simulink model "P2_SIL_Model_Diag"  (R2016a)
settings: Solver=ode2  StartTime=0.0  StopTime=Cycle_End  RelTol=1e-3
undefined symbols (not defined in the file): air, APP1_OOR, APP2_OOR, APP_Conversion_IN, APP_Mismatch, bms_inletair_temp, bms_maxchargecurrent, bms_maxdischargecurrent, BMS_Notfallkuehlung, BPP_Flt, cal, clt, ClutchEngag, CrankRequest, dcdc, eng, Engine, EngOverTemp, ENGTRQ_MSMCH_Degraded_CP, ENGTRQ_MSMCH_ErrCritical_CP, ENGTRQ_MSMCH_LimpHome_CP, EngTrqMismatch, env, ess, ESS, ESSOverTemp, fd, FFD, g, gb, Grade, IMG, KeyPos_Flt, KeyPosition, lib_APP_Conversion_IN, lib_ESS_plant_V1_2, lib_OBC_Manager, LossCAN, max_vehicle_rad_air_flow, MCUOverTemp, mot, MotDirMismatch, MotOverTemp, MotTrqMismatch, mph2kph, mph2ms, NeutralGear, obc, OBC_Manager, ParkGear, PRNDL_Flt, ReverseGear, RFD, rho, ShiftLeverPosition, sigbuilder_block, Speed, t_amb, time, tloop ... (+2)
libraries: simulink x104, EC2_libraries x12, Diagnostic x11, lib_CANerror_Detect x3, Utility x1
(part 9 of 11)

== system P2_SIL_Model_Diag/Controller/HSC/Powertrain Manager/Torque Distribution/Supervisory  Control  Logic1/VehReady.Transition.SyncCtrl ==
  EngSpeed : Inport
  MotorSpeed : Inport  Port=2
  f : TriggerPort  TriggerType=function-call  VariantControl=Variant
      settings: CopyFcn=Stateflow.SLINSF.SimulinkMan.removeBlockPreDeleteFcn  PreDeleteFcn=Stateflow.SLINSF.SimulinkMan.unsafePredeleteFcn
  Kp : Gain  Gain=1/100
  Saturation : Saturate  UpperLimit=20  LowerLimit=0
  Scope : Scope  NumInputPorts=2
  Sum : Sum  Inputs=|+-
  EngApp : Outport
  wires:
  MotorSpeed/1 -> Scope/1, Sum/1  "RPM"
  EngSpeed/1 -> Scope/2, Sum/2
  Sum/1 -> Kp/1
  Kp/1 -> Saturation/1
  Saturation/1 -> EngApp/1

== system P2_SIL_Model_Diag/Controller/HSC/Powertrain Manager/Torque Distribution/Supervisory  Control  Logic1/VehReady.Transition1.SyncCtrl ==
  EngSpeed : Inport
  MotorSpeed : Inport  Port=2
  f : TriggerPort  TriggerType=function-call  VariantControl=Variant
      settings: CopyFcn=Stateflow.SLINSF.SimulinkMan.removeBlockPreDeleteFcn  PreDeleteFcn=Stateflow.SLINSF.SimulinkMan.unsafePredeleteFcn
  Kp : Gain  Gain=1/100
  Saturation : Saturate  UpperLimit=20  LowerLimit=0
  Sum : Sum  Inputs=|+-
  EngApp : Outport
  wires:
  MotorSpeed/1 -> Sum/1  "RPM"
  EngSpeed/1 -> Sum/2
  Sum/1 -> Kp/1
  Kp/1 -> Saturation/1
  Saturation/1 -> EngApp/1

== system P2_SIL_Model_Diag/Controller/HSC/Powertrain Manager/Torque Distribution/Supervisory  Control  Logic1/VehReady.Transition2.SyncCtrl ==
  EngSpeed : Inport
  MotorSpeed : Inport  Port=2
  f : TriggerPort  TriggerType=function-call  VariantControl=Variant
      settings: CopyFcn=Stateflow.SLINSF.SimulinkMan.removeBlockPreDeleteFcn  PreDeleteFcn=Stateflow.SLINSF.SimulinkMan.unsafePredeleteFcn
  Kp : Gain  Gain=1/100
  Saturation : Saturate  UpperLimit=20  LowerLimit=0
  Sum : Sum  Inputs=|+-
  EngApp : Outport
  wires:
  MotorSpeed/1 -> Sum/1  "RPM"
  EngSpeed/1 -> Sum/2
  Sum/1 -> Kp/1
  Kp/1 -> Saturation/1
  Saturation/1 -> EngApp/1

== system P2_SIL_Model_Diag/Controller/HSC/Powertrain Manager/Torque Distribution/SysPwrMd ==
  SysPwrMd : Inport
  EngRunAtv : Inport  Port=2
  EngOnReq : Inport  Port=3
  Constant1 : Constant  Value=3
  Constant2 : Constant
  Saturation2 : Saturate  UpperLimit=2  LowerLimit=0
  Saturation3 : Saturate  UpperLimit=2  LowerLimit=0
  Switch1 : Switch  Threshold=1
  Switch2 : Switch  Threshold=1
  Switch3 : Switch  Threshold=1
  Out1 : Outport
  wires:
  Switch2/1 -> Switch3/3
  Constant1/1 -> Switch1/3
  Constant2/1 -> Switch2/1
  EngRunAtv/1 -> Switch2/2, Switch1/2
  Saturation2/1 -> Switch1/1
  SysPwrMd/1 -> Saturation3/1, Saturation2/1
  Saturation3/1 -> Switch2/3
  EngOnReq/1 -> Switch3/2
  Switch1/1 -> Switch3/1
  Switch3/1 -> Out1/1

== system P2_SIL_Model_Diag/Sensors/CAN/EBCAN/BMS_Antrieb/ISO_Hybrid_01_Resp ==
  Bus Creator : BusCreator  Inputs=3
  Constant : Constant  Value=100
  Constant1 : Constant  Value=100
  Constant2 : Constant  Value=100
  Out1 : Outport
  wires:
  Bus Creator/1 -> Out1/1  "ISO_Hybrid_01_Resp_Data"
  Constant2/1 -> Bus Creator/3  "ISO_Hybrid_01_Resp_Data_byte_5"
  Constant1/1 -> Bus Creator/2  "ISO_Hybrid_01_Resp_Data_byte_4"
  Constant/1 -> Bus Creator/1  "ISO_Hybrid_01_Resp_Data_byte_3"

== system P2_SIL_Model_Diag/Sensors/CAN/EBCAN/BMS_Antrieb/NMH_BMS ==
  In1 : Inport
  Bus Creator : BusCreator  Inputs=5
  Bus Selector : BusSelector  OutputSignals=NMH_BMS_Car_WakeUp,NMH_BMS_Normal_Mode_1,NMH_BMS_Normal_Mode_2,NMH_BMS_Start_1,NMH_BMS_Start_2
  Out1 : Outport
  wires:
  Bus Selector/1 -> Bus Creator/1  "<NMH_BMS_Car_WakeUp>"
  Bus Selector/2 -> Bus Creator/2  "<NMH_BMS_Normal_Mode_1>"
  Bus Selector/3 -> Bus Creator/3  "<NMH_BMS_Normal_Mode_2>"
  Bus Selector/4 -> Bus Creator/4  "<NMH_BMS_Start_1>"
  Bus Selector/5 -> Bus Creator/5  "<NMH_BMS_Start_2>"
  Bus Creator/1 -> Out1/1  "NMH_BMS"
  In1/1 -> Bus Selector/1

== system P2_SIL_Model_Diag/Sensors/CAN/EBCAN/CCM/ISO_Hybrid_01_Resp ==
  Bus Creator : BusCreator  Inputs=3
  Constant : Constant
  Constant1 : Constant
  Constant2 : Constant
  Out1 : Outport
  wires:
  Constant/1 -> Bus Creator/1  "ISO_Hybrid_01_Resp_Data_byte_3"
  Constant1/1 -> Bus Creator/2  "ISO_Hybrid_01_Resp_Data_byte_4"
  Constant2/1 -> Bus Creator/3  "ISO_Hybrid_01_Resp_Data_byte_5"
  Bus Creator/1 -> Out1/1  "ISO_Hybrid_01_Resp_Data"

== system P2_SIL_Model_Diag/Sensors/CAN/EBCAN/CCM/NMH_BMS ==
  Bus Creator : BusCreator  Inputs=5
  Constant{,1..4} (5 alike) : Constant
  Out1 : Outport
  wires:
  Bus Creator/1 -> Out1/1  "NMH_BMS"
  Constant4/1 -> Bus Creator/5  "NMH_BMS_Start_2"
  Constant3/1 -> Bus Creator/4  "NMH_BMS_Start_1"
  Constant2/1 -> Bus Creator/3  "NMH_BMS_Normal_Mode_2"
  Constant1/1 -> Bus Creator/2  "NMH_BMS_Normal_Mode_1"
  Constant/1 -> Bus Creator/1  "NMH_BMS_Car_WakeUp"

== system P2_SIL_Model_Diag/Sensors/CAN/EBCAN/ECM/ETEI_Engine_Torque_Status ==
  In1 : Inport
  Out1 : Outport
  wires:
  In1/1 -> Out1/1  "EngActStdyStTorq"

== system P2_SIL_Model_Diag/Sensors/CAN/EBCAN/ECM/PPEI_Vehicle_Speed_and_Distance ==
  In1 : Inport
  Out1 : Outport
  wires:
  In1/1 -> Out1/1  "VehSpdAvgDrvn"

== system P2_SIL_Model_Diag/Sensors/CAN/HV_CAN/BMS_Hybrid/BMS_HYB_02 ==
  In1 : Inport
  Bus Creator : BusCreator  Inputs=10
  Bus Selector : BusSelector  OutputSignals=BMS_Fehler_HS_offen,BMS_Fehler_Pilot,BMS_Init_abgescholssen,BMS_IstModus,BMS_IstSpannung,BMS_IstStrom,BMS_SleepInd,BMS_Fehler_Isolation,BMS_Fehler_HVBattAbschaltung,MO_BMS_Sollmodus
  Out1 : Outport
  wires:
  Bus Selector/1 -> Bus Creator/1  "<BMS_Fehler_HS_offen>"
  Bus Selector/2 -> Bus Creator/2  "<BMS_Fehler_Pilot>"
  Bus Selector/3 -> Bus Creator/3  "<BMS_Init_abgescholssen>"
  Bus Selector/4 -> Bus Creator/4  "<BMS_IstModus>"
  Bus Selector/5 -> Bus Creator/5  "<BMS_IstSpannung>"
  Bus Selector/6 -> Bus Creator/6  "<BMS_IstStrom>"
  Bus Selector/7 -> Bus Creator/7  "<BMS_SleepInd>"
  Bus Creator/1 -> Out1/1  "BMS_HYB_02"
  In1/1 -> Bus Selector/1
  Bus Selector/8 -> Bus Creator/8  "<BMS_Fehler_Isolation>"
  Bus Selector/9 -> Bus Creator/9  "<BMS_Fehler_HVBattAbschaltung>"
  Bus Selector/10 -> Bus Creator/10  "<MO_BMS_Sollmodus>"

== system P2_SIL_Model_Diag/Sensors/CAN/HV_CAN/BMS_Hybrid/BMS_HYB_03 ==
  In1 : Inport
  Bus Selector : BusSelector  OutputSignals=BMS_SOC
  Out1 : Outport
  wires:
  Bus Selector/1 -> Out1/1  "<BMS_SOC>"
  In1/1 -> Bus Selector/1

== system P2_SIL_Model_Diag/Sensors/CAN/HV_CAN/BMS_Hybrid/BMS_HYB_04 ==
  In1 : Inport
  Bus Selector : BusSelector  OutputSignals=BMS_Spannung_ZwKr
  Out1 : Outport
  wires:
  In1/1 -> Bus Selector/1  "BMS_Spannung_ZwKr"
  Bus Selector/1 -> Out1/1  "<BMS_Spannung_ZwKr>"

== system P2_SIL_Model_Diag/Sensors/CAN/HV_CAN/MCU/M165_Motor_Position_Info ==
  In1 : Inport
  Out1 : Outport
  wires:
  In1/1 -> Out1/1  "D2_Motor_Speed"

== system P2_SIL_Model_Diag/Sensors/CAN/HV_CAN/MCU/M166_Current_Info ==
  In1 : Inport
  Out1 : Outport
  wires:
  In1/1 -> Out1/1  "D4_DC_Bus_Current"

== system P2_SIL_Model_Diag/Sensors/CAN/HV_CAN/MCU/M167_Voltage_Info ==
  In1 : Inport
  Out1 : Outport
  wires:
  In1/1 -> Out1/1  "D1_DC_Bus_Voltage"

== system P2_SIL_Model_Diag/Sensors/CAN/HV_CAN/MCU/M170_Internal_States ==
  In1 : Inport
  Out1 : Outport
  wires:
  In1/1 -> Out1/1  "D6_Inverter_Enable_State"

== system P2_SIL_Model_Diag/Sensors/CAN/HV_CAN/MCU/M172_Torque_And_Timer_Info ==
  In1 : Inport
  Out1 : Outport
  wires:
  In1/1 -> Out1/1  "D2_Torque_Feedback"

== system P2_SIL_Model_Diag/Sensors/CAN/HV_CAN/MCU/M192_Command_Message ==
  In1 : Inport
  Out1 : Outport
  wires:
  In1/1 -> Out1/1  "Torque_Command"

== system P2_SIL_Model_Diag/Sensors/CAN/VEH_CAN/BCM/PPEI_Brake_Apply_Status ==
  In1 : Inport
  Out1 : Outport
  wires:
  In1/1 -> Out1/1  "BrkPdlPos"

== system P2_SIL_Model_Diag/Sensors/CAN/VEH_CAN/BCM/PPEI_Platfrom_General_Status ==
  In1 : Inport
  Out1 : Outport
  wires:
  In1/1 -> Out1/1  "SysPwrMd"

== system P2_SIL_Model_Diag/Sensors/CAN/VEH_CAN/EBCM/PPEI_Chassis_General_Status_1 ==
  Constant : Constant
  Out1 : Outport
  wires:
  Constant/1 -> Out1/1  "BrkPdlDrvAppPrsDetcd"

== system P2_SIL_Model_Diag/Camaro Plant Model/ESS/Soft BMS/Limits/Average Current/60 sec rolling average1 ==
  Instant : Inport
  1 second : Delay  DelayLength=1/tloop  InputProcessing=Inherited  SampleTime=tloop
  1sec trigger : Subsystem
  60 sec average : Subsystem
  Gain1 : Gain  Gain=tloop
  Sum1 : Sum  Inputs=++-
  accumulate : Memory  InheritSampleTime=on
  accumulate1 : Memory  InheritSampleTime=on
  Average : Outport
  wires:
  accumulate1/1 -> Average/1
  60 sec average/1(Average) -> accumulate1/1
  accumulate/1 -> Sum1/1
  1 second/1 -> Sum1/3
  Instant/1 -> Sum1/2, 1 second/1
  Sum1/1 -> Gain1/1, accumulate/1
  1sec trigger/1(Trigger) -> 60 sec average/Enable
  Gain1/1 -> 60 sec average/1(1sec)

== system P2_SIL_Model_Diag/Camaro Plant Model/ESS/Soft BMS/Limits/Average Current/60 sec rolling average2 ==
  Instant : Inport
  1 second : Delay  DelayLength=1/tloop  InputProcessing=Inherited  SampleTime=tloop
  1sec trigger : Subsystem
  60 sec average : Subsystem
  Gain1 : Gain  Gain=tloop
  Sum1 : Sum  Inputs=++-
  accumulate : Memory  InheritSampleTime=on
  accumulate1 : Memory  InheritSampleTime=on
  Average : Outport
  wires:
  Sum1/1 -> accumulate/1, Gain1/1
  Instant/1 -> 1 second/1, Sum1/2
  1 second/1 -> Sum1/3
  accumulate/1 -> Sum1/1
  60 sec average/1(Average) -> accumulate1/1
  accumulate1/1 -> Average/1
  1sec trigger/1(Trigger) -> 60 sec average/Enable
  Gain1/1 -> 60 sec average/1(1sec)

== system P2_SIL_Model_Diag/Camaro Plant Model/ICE Simple1/Engine Plant Modified/Core Engine/EngEfficiency/Divide by Zero Fix ==
  Multiply : Inport
  Divide : Inport  Port=2
  Compare To Zero : simulink/Logic and Bit Operations/Compare To Zero  relop===  OutDataTypeStr=boolean
  Constant1 : Constant  Value=0
  Constant2 : Constant
  Product2 : Product  Inputs=/*  SaturateOnIntegerOverflow=on  InputSameDT=on  OutDataTypeStr=Inherit: Same as first input
  Switch : Switch  Threshold=1
  Switch1 : Switch  Threshold=1
  Output : Outport
  wires:
  Multiply/1 -> Product2/2
  Switch1/1 -> Output/1
  Constant1/1 -> Switch1/1
  Product2/1 -> Switch1/3
  Switch/1 -> Product2/1
  Divide/1 -> Switch/3, Compare To Zero/1
  Constant2/1 -> Switch/1
  Compare To Zero/1 -> Switch1/2, Switch/2

== system P2_SIL_Model_Diag/Camaro Plant Model/IMG/IMG Plant/Clutch/Speed Calculaion/Clutch Accel ==
  y : Inport
  x : Inport  Port=2
  Mux : Mux  Inputs=2
  Switch : Switch  Threshold=0.5  SaturateOnIntegerOverflow=on  InputSameDT=on
  Zero : Constant  Value=0
  Zero check : RelationalOperator  Operator=~=  InputSameDT=on
  divide : Fcn  Expr=u[1]/u[2]
  eps : Constant  Value=eps
  x\y : Outport
  wires:
  Mux/1 -> divide/1
  x/1 -> Mux/1
  divide/1 -> x\y/1
  y/1 -> Zero check/1, Switch/1
  Zero/1 -> Zero check/2
  Zero check/1 -> Switch/2
  Switch/1 -> Mux/2
  eps/1 -> Switch/3

== system P2_SIL_Model_Diag/Camaro Plant Model/IMG/IMG Plant/Clutch/Speed Calculaion/Slip speed integrator ==
  Integrand : Inport
  Control : Inport  Port=2
  Reset value : Inport  Port=3
  Equal? : RelationalOperator  Operator===  InputSameDT=on
  IC : InitialCondition  Value=init
  Integrator : Integrator  ExternalReset=either  InitialConditionSource=external  LimitOutput=on  LowerSaturationLimit=0  AbsoluteTolerance=1e-3
  Switch : Switch  Threshold=0.5  SaturateOnIntegerOverflow=on  InputSameDT=on
  Switch1 : Switch  Threshold=0.5  SaturateOnIntegerOverflow=on  InputSameDT=on
  Zero : Constant  Value=0  OutDataTypeStr=boolean
  Zero1 : Constant  Value=0
  Output : Outport
  wires:
  IC/1 -> Integrator/3
  Integrand/1 -> Switch/1
  Switch/1 -> Integrator/1
  Equal?/1 -> Switch/2, Integrator/2, Switch1/2
  Zero1/1 -> Switch/3
  Zero/1 -> Equal?/2
  Integrator/1 -> Switch1/1
  Reset value/1 -> IC/1, Switch1/3
  Control/1 -> Equal?/1
  Switch1/1 -> Output/1

== system P2_SIL_Model_Diag/Camaro Plant Model/IMG/IMG Plant/Clutch/Speed Calculaion/input shaft free wheeling losses ==
  input shaft speed : Inport
  Constant1 : Constant  Value=0
  Fcn1 : Fcn  Expr=u==0
  Gain1 : Gain  Gain=0.08  SaturateOnIntegerOverflow=on  OutDataTypeStr=Inherit: Same as input  ParamDataTypeStr=Inherit: Same as input
  Switch2 : Switch  Threshold=0.5  SaturateOnIntegerOverflow=on  InputSameDT=on
  input shaft decel : Outport
  wires:
  input shaft speed/1 -> Switch2/3, Fcn1/1
  Fcn1/1 -> Switch2/2
  Gain1/1 -> input shaft decel/1
  Switch2/1 -> Gain1/1
  Constant1/1 -> Switch2/1

== system P2_SIL_Model_Diag/Camaro Plant Model/IMG/IMG Plant/Electric Machine/Calculate Mot Efficiency, MotPwrMech, and, MotPwrElec/Lower Limit ==
  In1 : Inport
  Constant3 : Constant  Value=Lolimit
  MinMax : MinMax  Function=max  Inputs=2
  Out1 : Outport
  wires:
  In1/1 -> MinMax/1
  Constant3/1 -> MinMax/2
  MinMax/1 -> Out1/1

== system P2_SIL_Model_Diag/Camaro Plant Model/IMG/IMG Plant/Electric Machine/MotTrqExcessTrigger/Signal Builder ==
  Demux : Demux  Tag=STV Demux  Outputs=1
  FromWs : FromWorkspace  Tag=STV FromWs  VariableName=tuvar  SampleTime=0
      SigBuilderData=|
      | common.afterFinalStr = 'Extrapolate'
      | common.sampleTime = 0
      | dataSet.timeRange = [0 521]
      | dataSet.name = 'Group 1'
      | sbobj.Groups.Name = 'Group 1'
      | sbobj.Groups.Signals.Name = 'Signal 1'
      | sbobj.Groups.Signals.XData = [0 75 100 220 245 521]
      | sbobj.Groups.Signals.YData = [0 0 0 0 0 0]
      | sbobj.Groups.TimeRange = [0 521]
  Signal 1 : Outport  Tag=STV Outport
  wires:
  Demux/1 -> Signal 1/1
  FromWs/1 -> Demux/1

== system P2_SIL_Model_Diag/Camaro Plant Model/IMG/IMG Plant/Electric Machine/Torque Calculation/electric machine filter ==
  trq : Inport
  Interval Test : simulink/Logic and Bit Operations/Interval Test  IntervalClosedRight=on  uplimit=0.02  IntervalClosedLeft=on  lowlimit=-0.02  OutDataTypeStr=boolean
  Switch : Switch  Threshold=0.5
  electric machine time response : TransferFcn  Denominator=[mot.plant.init.time_response 1]
  filtered : Outport
  wires:
  electric machine time response/1 -> Switch/3
  Interval Test/1 -> Switch/2
  trq/1 -> Interval Test/1, electric machine time response/1, Switch/1
  Switch/1 -> filtered/1

== system P2_SIL_Model_Diag/Camaro Plant Model/IMG/IMG Plant/Electric Machine/Torque Calculation/max torque  ==
  cmd : Inport
  speed : Inport  Port=2
  Memory : Memory
  Peak trq max - Motoring : Lookup  InputValues=mot.plant.init.regen.trq_max.idx1_spd  Table=mot.plant.init.motor.trq_max.map  LookUpMeth=Interpolation-Use End Values  SaturateOnIntegerOverflow=on
  Peak trq max - Regen : Lookup  InputValues=mot.plant.init.regen.trq_max.idx1_spd  Table=mot.plant.init.regen.trq_max.map  LookUpMeth=Interpolation-Use End Values  SaturateOnIntegerOverflow=on
  Switch1 : Switch  SaturateOnIntegerOverflow=on
  rad/s  to RPM : Gain  Gain=30/pi
  max torque : Outport
  wires:
  Peak trq max - Regen/1 -> Switch1/3
  Peak trq max - Motoring/1 -> Switch1/1
  speed/1 -> rad/s  to RPM/1
  cmd/1 -> Switch1/2
  Switch1/1 -> max torque/1
  Memory/1 -> Peak trq max - Motoring/1, Peak trq max - Regen/1
  rad/s  to RPM/1 -> Memory/1

== system P2_SIL_Model_Diag/Camaro Plant Model/IMG/Soft MCU/Torque Calculation/max torque /Divide by zero ==
  In1 : Inport
  Compare To Constant : simulink/Logic and Bit Operations/Compare To Constant  relop===  const=0  OutDataTypeStr=boolean
  Constant1 : Constant
  Switch2 : Switch  Criteria=u2 > Threshold
  Out1 : Outport
  wires:
  Constant1/1 -> Switch2/1
  Compare To Constant/1 -> Switch2/2
  In1/1 -> Switch2/3, Compare To Constant/1
  Switch2/1 -> Out1/1

== system P2_SIL_Model_Diag/Camaro Plant Model/IMG/Soft MCU/Torque Calculation/max torque /Heat index ==
  note: Heat index calculation
  cont torque : Inport
  torque : Inport  Port=2
  Abs : Abs  SaturateOnIntegerOverflow=on
  Divide : Subsystem  mask(Divide){}
      mask Display: disp('Divide')
  Heat Energy Factor : Integrator  InitialCondition=-0.3  LimitOutput=on  UpperSaturationLimit=1  LowerSaturationLimit=-0.3
  Heating Constant : Gain  Gain=0.3/mot.plant.init.t_max_trq  SaturateOnIntegerOverflow=on  OutDataTypeStr=Inherit: Same as input  ParamDataTypeStr=Inherit: Same as input
  Saturation : Saturate  UpperLimit=1  LowerLimit=0
  Sum : Sum  Inputs=+-  SaturateOnIntegerOverflow=on  InputSameDT=on  OutDataTypeStr=Inherit: Same as first input
  motor inertia (Nms^2\rad)5 : Constant
  Heat index : Outport
  wires:
  cont torque/1 -> Divide/2(denominator)
  Abs/1 -> Sum/1
  Saturation/1 -> Heat index/1
  motor inertia (Nms^2\rad)5/1 -> Sum/2
  Divide/1(quotient) -> Abs/1
  Sum/1 -> Heating Constant/1
  Heating Constant/1 -> Heat Energy Factor/1
  Heat Energy Factor/1 -> Saturation/1
  torque/1 -> Divide/1(numerator)

== system P2_SIL_Model_Diag/Camaro Plant Model/Transmission1/Transmission Plant/Gearbox/Speed Calculation/P//N ==
  torque input : Inport
  Inertia Input : Inport  Port=2
  gear : Inport  Port=3
  inital speed : Inport  Port=4
  (0,inf) : Saturate  UpperLimit=inf  LowerLimit=0
  Fcn2 : Fcn  Expr=u==0
  Integrator : Integrator  ExternalReset=rising  InitialConditionSource=external
  Memory : Memory
  Subsystem2 : Subsystem
      mask Display: disp('divider')
  Sum : Sum  Inputs=-+|  SaturateOnIntegerOverflow=on  InputSameDT=on  OutDataTypeStr=Inherit: Same as first input
  input shaft free wheeling losses : Subsystem
  speed : Outport
  wires:
  Inertia Input/1 -> Subsystem2/2(In2)
  Fcn2/1 -> Integrator/2
  Subsystem2/1(Out1) -> Integrator/1
  Memory/1 -> Integrator/3
  (0,inf)/1 -> speed/1
  gear/1 -> Fcn2/1
  inital speed/1 -> Memory/1
  torque input/1 -> Sum/2
  Sum/1 -> Subsystem2/1(In1)
  input shaft free wheeling losses/1(input shaft decel) -> Sum/1
  Integrator/1 -> input shaft free wheeling losses/1(input shaft speed), (0,inf)/1

== system P2_SIL_Model_Diag/Camaro Plant Model/Transmission1/Transmission Plant/Gearbox/Speed Calculation/R//D ==
  spd in : Inport
  gear number : Inport  Port=2
  Constant5 : Constant
  Constant6 : Constant  Value=gb.plant.init.shift_time
  Integrator : Integrator  ExternalReset=rising
  Relational Operator4 : RelationalOperator  Operator=~=  InputSameDT=on
  Relational Operator5 : RelationalOperator  Operator=<=  InputSameDT=on
  S-R Flip-Flop : Subsystem  mask(SRFlipFlop){initial_condition=0}
      mask prompts: initial_condition "Initial condition:"
      mask help: S-R Flip Flop Block
  Switch : Switch  Threshold=0.5  SaturateOnIntegerOverflow=on  InputSameDT=on
  Transfer Fcn : TransferFcn  Denominator=[.2 1]
  Unit Delay7 : Memory
  term2 : Terminator
  spd in filtered : Outport
  wires:
  Transfer Fcn/1 -> Switch/1
  Switch/1 -> spd in filtered/1
  Relational Operator5/1 -> S-R Flip-Flop/2(R)
  S-R Flip-Flop/1(Q) -> Switch/2
  Integrator/1 -> Relational Operator5/2
  Relational Operator4/1 -> S-R Flip-Flop/1(S), Integrator/2
  Unit Delay7/1 -> Relational Operator4/2
  S-R Flip-Flop/2(!Q) -> term2/1
  Constant6/1 -> Relational Operator5/1
  Constant5/1 -> Integrator/1
  spd in/1 -> Transfer Fcn/1, Switch/3
  gear number/1 -> Unit Delay7/1, Relational Operator4/1

== system P2_SIL_Model_Diag/Camaro Plant Model/Transmission1/Transmission Plant/Gearbox/Torque calculation/Blending (state dependent) ==
  Input : Inport
  Control (state) : Inport  Port=2
  Linear spline : Fcn  Expr=(u<xl)*yl + (xl<=u)*(u<xc)*((yc-yl)*(u-xl)/(xc-xl)+yl) + (xc<=u)*(u<xr)*((yc-yr)*(u-xr)/(xc-xr)+yr) + (xr<=u)*yr
  Product2 : Product  SaturateOnIntegerOverflow=on  InputSameDT=on  OutDataTypeStr=Inherit: Same as first input
  Output : Outport
  wires:
  Control (state)/1 -> Linear spline/1
  Product2/1 -> Output/1
  Linear spline/1 -> Product2/2
  Input/1 -> Product2/1

== system P2_SIL_Model_Diag/Camaro Plant Model/Transmission1/Transmission Plant/Torque Converter/Speed Calculation/Pump Accel ==
  y : Inport
  x : Inport  Port=2
  Mux : Mux  Inputs=2
  Switch : Switch  Threshold=0.5  SaturateOnIntegerOverflow=on  InputSameDT=on
  Zero : Constant  Value=0
  Zero check : RelationalOperator  Operator=~=  InputSameDT=on
  divide : Fcn  Expr=u[1]/u[2]
  eps : Constant  Value=eps
  x\y : Outport
  wires:
  eps/1 -> Switch/3
  Switch/1 -> Mux/2
  Zero check/1 -> Switch/2
  Zero/1 -> Zero check/2
  y/1 -> Switch/1, Zero check/1
  divide/1 -> x\y/1
  x/1 -> Mux/1
  Mux/1 -> divide/1

== system P2_SIL_Model_Diag/Camaro Plant Model/Transmission1/Transmission Plant/Torque Converter/Speed Calculation/Slip speed integrator ==
  note: torque converter locked => spd in = spd out
      | when unlocked, spd in = integral of (Tin-Tloss)\J
  Integral : Inport
  Control : Inport  Port=2
  Reset value : Inport  Port=3
  Equal? : RelationalOperator  Operator===  OutDataTypeStr=boolean  InputSameDT=on
  IC : InitialCondition  Value=init
  Integrator : Integrator  ExternalReset=either  InitialConditionSource=external  LimitOutput=on  LowerSaturationLimit=0  AbsoluteTolerance=1e-3
  Switch : Switch  Threshold=0.5  SaturateOnIntegerOverflow=on  InputSameDT=on
  Switch1 : Switch  Threshold=0.5  SaturateOnIntegerOverflow=on  InputSameDT=on
  Zero : Constant  Value=0  OutDataTypeStr=boolean
  Zero1 : Constant  Value=0
  Output : Outport
  wires:
  Reset value/1 -> Switch1/3, IC/1
  Switch1/1 -> Output/1
  Integrator/1 -> Switch1/1
  Zero/1 -> Equal?/2
  Zero1/1 -> Switch/3
  Equal?/1 -> Switch1/2, Integrator/2, Switch/2
  Switch/1 -> Integrator/1
  Integral/1 -> Switch/1
  Control/1 -> Equal?/1
  IC/1 -> Integrator/3

== system P2_SIL_Model_Diag/Camaro Plant Model/Transmission1/Transmission Plant/Torque Converter/Torque Calculation/ Hydraulic Dynamic Torque ==
  input_trq : Inport
  Rt : Inport  Port=2
  Rw : Inport  Port=3
  impeller_spd : Inport  Port=4
  Divide : Product  Inputs=*/
  K Factor : Lookup  InputValues=tc.plant.init.k_factor.idx1_spd_ratio  Table=tc.plant.init.k_factor.map  LookUpMeth=Interpolation-Use End Values  SaturateOnIntegerOverflow=on
  Product1 : Product  SaturateOnIntegerOverflow=on  InputSameDT=on  OutDataTypeStr=Inherit: Same as first input
  Product2 : Product  SaturateOnIntegerOverflow=on  InputSameDT=on  OutDataTypeStr=Inherit: Same as first input
  Product3 : Product  SaturateOnIntegerOverflow=on  InputSameDT=on  OutDataTypeStr=Inherit: Same as first input
  Sum : Sum  Inputs=-+
  turbine_trq : Outport
  impeller_trq : Outport  Port=2
  wires:
  Product1/1 -> Divide/2  "K^2"
  Product3/1 -> turbine_trq/1  "Tt_hd"
  Rt/1 -> Product3/1
  input_trq/1 -> Sum/2
  Sum/1 -> impeller_trq/1
  impeller_spd/1 -> Product2/2, Product2/1
  Product2/1 -> Divide/1  "Wi^2"
  Divide/1 -> Product3/2, Sum/1  "Ti_hd"
  K Factor/1 -> Product1/1, Product1/2  "K"
  Rw/1 -> K Factor/1

== system P2_SIL_Model_Diag/Camaro Plant Model/Transmission1/Transmission Plant/Torque Converter/Torque Calculation/spd and trq ratio ==
  impeller spd : Inport
  turbine spd : Inport  Port=2
  Torque Ratio : Lookup  InputValues=tc.plant.init.spd_ratio  Table=tc.plant.init.trq_ratio  LookUpMeth=Interpolation-Use End Values  SaturateOnIntegerOverflow=on
  speed ratio : Subsystem  mask(Divider){}
      mask help: Divide input 1 by input 2.
      mask Help:
      | This block implements a divider; division by zero is taken care of in the following manner:
      | if u[2] equals 0,
      |    the output is u[1]/eps,
      | else
      |    the output is u[1]/u[2].
      mask Display: disp('/')
  Rt : Outport
  Rw : Outport  Port=2
  wires:
  Torque Ratio/1 -> Rt/1
  speed ratio/1(quotient) -> Rw/1, Torque Ratio/1
  impeller spd/1 -> speed ratio/2(denominator)
  turbine spd/1 -> speed ratio/1(numerator)

== system P2_SIL_Model_Diag/Controller/HSC/Camaro Fault Detection/Component Diagnostic/Engine Component Diagnostic/Override  engTrqCmd ==
  note: This subsystem is used to override the model value of a signal to a constant value
  note: Override Switch Subsystem
  In1 : Inport
  Constant : Constant  Value=50
  Multiport Switch : MultiPortSwitch  DataPortOrder=Zero-based contiguous  Inputs=2  zeroidx=on
  Signal Override Switch 0 = Use Model 1 = Use Constant : Constant
  Out1 : Outport
  wires:
  Signal Override Switch 0 = Use Model 1 = Use Constant/1 -> Multiport Switch/1
  In1/1 -> Multiport Switch/2
  Multiport Switch/1 -> Out1/1
  Constant/1 -> Multiport Switch/3

== system P2_SIL_Model_Diag/Controller/HSC/Camaro Fault Detection/Component Diagnostic/Engine Component Diagnostic/TorqMismatch Detection ==
  In1 : Inport
  In2 : Inport  Port=2
  In3 : Inport  Port=3
  Abs : Abs
  Add : Sum  Inputs=+-
  Bus Creator : BusCreator  Inputs=3
  Constant : Constant  Value=cal.ENGTRQ_MSMCH.ErrCritical_CP
  Constant1 : Constant  Value=50
  Constant2 : Constant  Value=cal.ENGTRQ_MSMCH.Degraded_CP
  Constant3 : Constant  Value=cal.ENGTRQ_MSMCH.LimpHome_CP
  Relational Operator : RelationalOperator  OutDataTypeStr=boolean
  Relational Operator1 : RelationalOperator  Operator=>  OutDataTypeStr=boolean
  Relational Operator2 : RelationalOperator  Operator=>  OutDataTypeStr=boolean
  Switch : Switch  Threshold=1
  Terminator : Terminator
  Unit Delay : UnitDelay  Commented=through  SampleTime=-1
  Unit Delay1 : UnitDelay  Commented=through  SampleTime=-1
  "Zero " : Constant  Value=0
  Eng_Torque_Mismch : Outport
  wires:
  In1/1 -> Unit Delay/1
  In2/1 -> Unit Delay1/1
  "Zero "/1 -> Switch/3
  In3/1 -> Switch/2
  Unit Delay/1 -> Add/1
  Constant/1 -> Relational Operator/2
  Add/1 -> Abs/1
  Relational Operator/1 -> Switch/1
  Switch/1 -> Bus Creator/1, Relational Operator2/1, Relational Operator1/1  "Eng_Torque_Mismch_Critical"
  Constant2/1 -> Relational Operator1/2
  Constant3/1 -> Relational Operator2/2
  Relational Operator1/1 -> Bus Creator/2  "Eng_Torque_Mismch_Degrad"
  Relational Operator2/1 -> Bus Creator/3  "Eng_Torque_Mismch_Limp"
  Bus Creator/1 -> Eng_Torque_Mismch/1
  Unit Delay1/1 -> Add/2
  Abs/1 -> Terminator/1
  Constant1/1 -> Relational Operator/1

== system P2_SIL_Model_Diag/Controller/HSC/Camaro Fault Detection/Component Diagnostic/Motor Component Diagnostic/MCU_ESS_Voltage_Mismatch ==
  MCU_Voltage : Inport
  ESS_Voltage : Inport  Port=2
  Abs : Abs
  Add : Sum  Inputs=-+
  Constant : Constant  Value=cal.Diag.MCU.ESSVLT_MSMCH
  Relational Operator : RelationalOperator  OutDataTypeStr=boolean
  MCU_ESS_Voltage_Mismch : Outport
  wires:
  Relational Operator/1 -> MCU_ESS_Voltage_Mismch/1
  Constant/1 -> Relational Operator/2
  Abs/1 -> Relational Operator/1
  ESS_Voltage/1 -> Add/2
  Add/1 -> Abs/1
  MCU_Voltage/1 -> Add/1

== system P2_SIL_Model_Diag/Controller/HSC/Camaro Fault Detection/Component Diagnostic/Motor Component Diagnostic/Motor_Direction_Mismatch ==
  note: 1: mismatch
      | 0: no failure
  Direction_Command : Inport
  Direction_Feedback : Inport  Port=2
  Inverter_enable_state : Inport  Port=3
  Logical Operator : Logic  AllPortsSameDT=off  OutDataTypeStr=boolean
  Relational Operator : RelationalOperator  Operator=~=  OutDataTypeStr=boolean
  Direction_Mismch : Outport
  wires:
  Relational Operator/1 -> Logical Operator/1
  Logical Operator/1 -> Direction_Mismch/1
  Direction_Command/1 -> Relational Operator/1  "Direction_Command"
  Direction_Feedback/1 -> Relational Operator/2  "Direction_Feedback"
  Inverter_enable_state/1 -> Logical Operator/2  "Inverter_enable_state"

== system P2_SIL_Model_Diag/Controller/HSC/Camaro Fault Detection/Component Diagnostic/Motor Component Diagnostic/Override  fault ==
  note: This subsystem is used to override the model value of a signal to a constant value
  note: Override Switch Subsystem
  In1 : Inport
  Multiport Switch : MultiPortSwitch  DataPortOrder=Zero-based contiguous  Inputs=2  zeroidx=on
  Override Value : Constant  Value=0  OutDataTypeStr=double
  Signal Override Switch 0 = Use Model 1 = Use Constant : Constant
  Out1 : Outport
  wires:
  Signal Override Switch 0 = Use Model 1 = Use Constant/1 -> Multiport Switch/1
  In1/1 -> Multiport Switch/2
  Multiport Switch/1 -> Out1/1
  Override Value/1 -> Multiport Switch/3

== system P2_SIL_Model_Diag/Controller/HSC/Camaro Fault Detection/Component Diagnostic/Motor Component Diagnostic/Override  fault1 ==
  note: Override Switch Subsystem
  note: This subsystem is used to override the model value of a signal to a constant value
  In1 : Inport
  Multiport Switch : MultiPortSwitch  DataPortOrder=Zero-based contiguous  Inputs=2  zeroidx=on
  Override Value : Constant  Value=0  OutDataTypeStr=double
  Signal Override Switch 0 = Use Model 1 = Use Constant : Constant  Value=0
  Out1 : Outport
  wires:
  Override Value/1 -> Multiport Switch/3
  Multiport Switch/1 -> Out1/1
  In1/1 -> Multiport Switch/2
  Signal Override Switch 0 = Use Model 1 = Use Constant/1 -> Multiport Switch/1

== system P2_SIL_Model_Diag/Controller/HSC/Camaro Fault Detection/Component Diagnostic/Motor Component Diagnostic/Torque_Mismatch ==
  MCU_torq_command : Inport
  Torq_feedback : Inport  Port=2
  Abs : Abs
  Abs1 : Abs
  Abs2 : Abs
  Add : Sum  Inputs=+-
  Bus Creator : BusCreator  Inputs=3
  Constant : Constant  Value=cal.MOTTRQ_MSMCH.ErrCritical_CP
  Constant1 : Constant  Value=cal.MOTTRQ_MSMCH.Degraded_CP
  Constant2 : Constant  Value=cal.MOTTRQ_MSMCH.LimpHome_CP
  Constant3 : Constant  Value=0
  Conversion  APP1 (%) : DataTypeConversion  OutDataTypeStr=boolean
  Latch : Subsystem
  Relational Operator : RelationalOperator  Operator=>  OutDataTypeStr=boolean
  Relational Operator1 : RelationalOperator  Operator=>  OutDataTypeStr=boolean
  Relational Operator2 : RelationalOperator  Operator=>  OutDataTypeStr=boolean
  Unit Delay : UnitDelay  SampleTime=-1
  MCU_Torque_Mismch : Outport
  wires:
  Unit Delay/1 -> Abs/1
  Abs/1 -> Add/1
  Torq_feedback/1 -> Abs1/1
  Abs1/1 -> Add/2
  MCU_torq_command/1 -> Unit Delay/1
  Constant/1 -> Relational Operator/2
  Constant1/1 -> Relational Operator1/2
  Constant2/1 -> Relational Operator2/2
  Relational Operator1/1 -> Bus Creator/2  "MCU_Torque_Mismch_Degrad"
  Relational Operator2/1 -> Bus Creator/3  "MCU_Torque_Mismch_Limp"
  Bus Creator/1 -> MCU_Torque_Mismch/1
  Add/1 -> Abs2/1
  Abs2/1 -> Relational Operator/1, Relational Operator2/1, Relational Operator1/1
  Constant3/1 -> Conversion  APP1 (%)/1
  Relational Operator/1 -> Latch/1(In1)  "MCU_Torque_Mismch_Critical"
  Latch/1(Out1) -> Bus Creator/1  "MCU_Torque_Mismch_Critical"
  Conversion  APP1 (%)/1 -> Latch/2(In2)

== system P2_SIL_Model_Diag/Controller/HSC/Camaro Fault Detection/Input Conversions/BMS_Conversions/BMS_rollingAliveCnt ==
  Constant : Constant
  Rolling Alive Counter : Stateflow chart  TreatAsAtomicUnit=on
  Switch : Switch  Criteria=u2 > Threshold
  Out1 : Outport
  wires:
  Switch/1 -> Out1/1  "BMS_rollingAliveCnt [0 1 2 3]"
  [BMS_CAN_fault] -> Switch/2
  Constant/1 -> Switch/1
  Rolling Alive Counter/1(RollingAliveCnt) -> Switch/3

== system P2_SIL_Model_Diag/Controller/HSC/Camaro Fault Detection/Input Conversions/BMS_Conversions/Override  BMS_gdf 0_1 ==
  note: Override Switch Subsystem
  note: This subsystem is used to override the model value of a signal to a constant value
  In1 : Inport
  Multiport Switch : MultiPortSwitch  DataPortOrder=Zero-based contiguous  Inputs=2  zeroidx=on
  Override Value : Constant  Value=0  OutDataTypeStr=double
  Signal Override Switch 0 = Use Model 1 = Use Constant : Constant
  Out1 : Outport
  wires:
  Override Value/1 -> Multiport Switch/3
  Multiport Switch/1 -> Out1/1
  In1/1 -> Multiport Switch/2
  Signal Override Switch 0 = Use Model 1 = Use Constant/1 -> Multiport Switch/1

== system P2_SIL_Model_Diag/Controller/HSC/Camaro Fault Detection/Input Conversions/BMS_Conversions/Override  closeContactorsCmd ==
  note: This subsystem is used to override the model value of a signal to a constant value
  note: Override Switch Subsystem
  In1 : Inport
  Multiport Switch : MultiPortSwitch  DataPortOrder=Zero-based contiguous  Inputs=2  zeroidx=on
  Override Value : Constant  Value=0  OutDataTypeStr=double
  Signal Override Switch 0 = Use Model 1 = Use Constant : Constant  Value=0
  Out1 : Outport
  wires:
  Signal Override Switch 0 = Use Model 1 = Use Constant/1 -> Multiport Switch/1
  In1/1 -> Multiport Switch/2
  Multiport Switch/1 -> Out1/1
  Override Value/1 -> Multiport Switch/3

== system P2_SIL_Model_Diag/Controller/HSC/Camaro Fault Detection/Input Conversions/BMS_Conversions/Override  contactorsClsd ==
  note: This subsystem is used to override the model value of a signal to a constant value
  note: Override Switch Subsystem
  In1 : Inport
  Multiport Switch : MultiPortSwitch  DataPortOrder=Zero-based contiguous  Inputs=2  zeroidx=on
  Override Value : Constant  Value=0  OutDataTypeStr=double
  Signal Override Switch 0 = Use Model 1 = Use Constant : Constant  Value=0
  Out1 : Outport
  wires:
  Signal Override Switch 0 = Use Model 1 = Use Constant/1 -> Multiport Switch/1
  In1/1 -> Multiport Switch/2
  Multiport Switch/1 -> Out1/1
  Override Value/1 -> Multiport Switch/3

== system P2_SIL_Model_Diag/Controller/HSC/Camaro Fault Detection/Input Conversions/BMS_Conversions/Override  essCur_A ==
  note: Override Switch Subsystem
  note: This subsystem is used to override the model value of a signal to a constant value
  In1 : Inport
  Multiport Switch : MultiPortSwitch  DataPortOrder=Zero-based contiguous  Inputs=2  zeroidx=on
  Override Value : Constant  Value=0  OutDataTypeStr=double
  Signal Override Switch 0 = Use Model 1 = Use Constant : Constant  Value=0
  Out1 : Outport
  wires:
  Override Value/1 -> Multiport Switch/3
  Multiport Switch/1 -> Out1/1
  In1/1 -> Multiport Switch/2
  Signal Override Switch 0 = Use Model 1 = Use Constant/1 -> Multiport Switch/1

== system P2_SIL_Model_Diag/Controller/HSC/Camaro Fault Detection/Input Conversions/BMS_Conversions/Override  essSOC_0_1 ==
  note: This subsystem is used to override the model value of a signal to a constant value
  note: Override Switch Subsystem
  In1 : Inport
  Multiport Switch : MultiPortSwitch  DataPortOrder=Zero-based contiguous  Inputs=2  zeroidx=on
  Override Value : Constant  Value=0  OutDataTypeStr=double
  Signal Override Switch 0 = Use Model 1 = Use Constant : Constant  Value=0
  Out1 : Outport
  wires:
  Signal Override Switch 0 = Use Model 1 = Use Constant/1 -> Multiport Switch/1
  In1/1 -> Multiport Switch/2
  Multiport Switch/1 -> Out1/1
  Override Value/1 -> Multiport Switch/3

== system P2_SIL_Model_Diag/Controller/HSC/Camaro Fault Detection/Input Conversions/BMS_Conversions/Override  essTemp_C ==
  note: This subsystem is used to override the model value of a signal to a constant value
  note: Override Switch Subsystem
  In1 : Inport
  Multiport Switch : MultiPortSwitch  DataPortOrder=Zero-based contiguous  Inputs=2  zeroidx=on
  Override Value : Constant  Value=0  OutDataTypeStr=double
  Signal Override Switch 0 = Use Model 1 = Use Constant : Constant
  Out1 : Outport
  wires:
  Signal Override Switch 0 = Use Model 1 = Use Constant/1 -> Multiport Switch/1
  In1/1 -> Multiport Switch/2
  Multiport Switch/1 -> Out1/1
  Override Value/1 -> Multiport Switch/3

== system P2_SIL_Model_Diag/Controller/HSC/Camaro Fault Detection/Input Conversions/BMS_Conversions/Override  hvBattVolt_V ==
  note: This subsystem is used to override the model value of a signal to a constant value
  note: Override Switch Subsystem
  In1 : Inport
  Multiport Switch : MultiPortSwitch  DataPortOrder=Zero-based contiguous  Inputs=2  zeroidx=on
  Override Value : Constant  Value=0  OutDataTypeStr=double
  Signal Override Switch 0 = Use Model 1 = Use Constant : Constant  Value=0
  Out1 : Outport
  wires:
  Signal Override Switch 0 = Use Model 1 = Use Constant/1 -> Multiport Switch/1
  In1/1 -> Multiport Switch/2
  Multiport Switch/1 -> Out1/1
  Override Value/1 -> Multiport Switch/3

== system P2_SIL_Model_Diag/Controller/HSC/Camaro Fault Detection/Input Conversions/BMS_Conversions/Override  hvBusVolt_V ==
  note: Override Switch Subsystem
  note: This subsystem is used to override the model value of a signal to a constant value
  In1 : Inport
  Multiport Switch : MultiPortSwitch  DataPortOrder=Zero-based contiguous  Inputs=2  zeroidx=on
  Override Value : Constant  Value=0  OutDataTypeStr=double
  Signal Override Switch 0 = Use Model 1 = Use Constant : Constant  Value=0
  Out1 : Outport
  wires:
  Override Value/1 -> Multiport Switch/3
  Multiport Switch/1 -> Out1/1
  In1/1 -> Multiport Switch/2
  Signal Override Switch 0 = Use Model 1 = Use Constant/1 -> Multiport Switch/1

== system P2_SIL_Model_Diag/Controller/HSC/Camaro Fault Detection/Input Conversions/BMS_Conversions/Override  rollingAliveCnt [1_3] ==
  note: Override Switch Subsystem
  note: This subsystem is used to override the model value of a signal to a constant value
  In1 : Inport
  Multiport Switch : MultiPortSwitch  DataPortOrder=Zero-based contiguous  Inputs=2  zeroidx=on
  Override Value : Constant  Value=0  OutDataTypeStr=double
  Signal Override Switch 0 = Use Model 1 = Use Constant : Constant  Value=0
  Out1 : Outport
  wires:
  Override Value/1 -> Multiport Switch/3
  Multiport Switch/1 -> Out1/1
  In1/1 -> Multiport Switch/2
  Signal Override Switch 0 = Use Model 1 = Use Constant/1 -> Multiport Switch/1

== system P2_SIL_Model_Diag/Controller/HSC/Camaro Fault Detection/Input Conversions/Clutch_Conversions/Clutch_Rolling ==
  Constant8 : Constant
  Rolling Alive Counter1 : Stateflow chart  TreatAsAtomicUnit=on
  Switch1 : Switch  Criteria=u2 > Threshold
  Out1 : Outport
  wires:
  [Clutch_CAN_fault] -> Switch1/2
  Rolling Alive Counter1/1(RollingAliveCnt) -> Switch1/3
  Constant8/1 -> Switch1/1
  Switch1/1 -> Out1/1  "ClutchRollingAliveCnt [0 1 2 3]"

== system P2_SIL_Model_Diag/Controller/HSC/Camaro Fault Detection/Input Conversions/Clutch_Conversions/Override  Engage_Clutch  ==
  note: This subsystem is used to override the model value of a signal to a constant value
  note: Override Switch Subsystem
  In1 : Inport
  Multiport Switch : MultiPortSwitch  DataPortOrder=Zero-based contiguous  Inputs=2  zeroidx=on
  Override Value : Constant  Value=0  OutDataTypeStr=double
  Signal Override Switch 0 = Use Model 1 = Use Constant : Constant
  Out1 : Outport
  wires:
  Signal Override Switch 0 = Use Model 1 = Use Constant/1 -> Multiport Switch/1
  In1/1 -> Multiport Switch/2
  Multiport Switch/1 -> Out1/1
  Override Value/1 -> Multiport Switch/3

== system P2_SIL_Model_Diag/Controller/HSC/Camaro Fault Detection/Input Conversions/Clutch_Conversions/Override  rollingAliveCnt [123] ==
  note: Override Switch Subsystem
  note: This subsystem is used to override the model value of a signal to a constant value
  In1 : Inport
  Multiport Switch : MultiPortSwitch  DataPortOrder=Zero-based contiguous  Inputs=2  zeroidx=on
  Override Value : Constant  Value=0  OutDataTypeStr=double
  Signal Override Switch 0 = Use Model 1 = Use Constant : Constant  Value=0
  Out1 : Outport
  wires:
  Override Value/1 -> Multiport Switch/3
  Multiport Switch/1 -> Out1/1
  In1/1 -> Multiport Switch/2
  Signal Override Switch 0 = Use Model 1 = Use Constant/1 -> Multiport Switch/1

== system P2_SIL_Model_Diag/Controller/HSC/Camaro Fault Detection/Input Conversions/DriverInput_Conversions/Override  KeyPos [0_3] ==
  note: Override Switch Subsystem
  note: This subsystem is used to override the model value of a signal to a constant value
  In1 : Inport
  Multiport Switch : MultiPortSwitch  DataPortOrder=Zero-based contiguous  Inputs=2  zeroidx=on
  Override Value : Constant  Value=0  OutDataTypeStr=double
  Signal Override Switch 0 = Use Model 1 = Use Constant : Constant  Value=0
  Out1 : Outport
  wires:
  Override Value/1 -> Multiport Switch/3
  Multiport Switch/1 -> Out1/1
  In1/1 -> Multiport Switch/2
  Signal Override Switch 0 = Use Model 1 = Use Constant/1 -> Multiport Switch/1

== system P2_SIL_Model_Diag/Controller/HSC/Camaro Fault Detection/Input Conversions/DriverInput_Conversions/Override APP (%) ==
  note: Override Switch Subsystem
  note: This subsystem is used to override the model value of a signal to a constant value
  In1 : Inport
  Multiport Switch : MultiPortSwitch  DataPortOrder=Zero-based contiguous  Inputs=2  zeroidx=on
  Override Value : Constant  Value=0  OutDataTypeStr=double
  Signal Override Switch 0 = Use Model 1 = Use Constant : Constant  Value=0
  Out1 : Outport
  wires:
  Override Value/1 -> Multiport Switch/3
  Multiport Switch/1 -> Out1/1
  In1/1 -> Multiport Switch/2
  Signal Override Switch 0 = Use Model 1 = Use Constant/1 -> Multiport Switch/1

== system P2_SIL_Model_Diag/Controller/HSC/Camaro Fault Detection/Input Conversions/DriverInput_Conversions/Override BPP (%) ==
  note: This subsystem is used to override the model value of a signal to a constant value
  note: Override Switch Subsystem
  In1 : Inport
  Multiport Switch : MultiPortSwitch  DataPortOrder=Zero-based contiguous  Inputs=2  zeroidx=on
  Override Value : Constant  Value=0  OutDataTypeStr=double
  Signal Override Switch 0 = Use Model 1 = Use Constant : Constant  Value=0
  Out1 : Outport
  wires:
  Signal Override Switch 0 = Use Model 1 = Use Constant/1 -> Multiport Switch/1
  In1/1 -> Multiport Switch/2
  Multiport Switch/1 -> Out1/1
  Override Value/1 -> Multiport Switch/3

== system P2_SIL_Model_Diag/Controller/HSC/Camaro Fault Detection/Input Conversions/DriverInput_Conversions/Override PRNDL ==
  note: Override Switch Subsystem
  note: This subsystem is used to override the model value of a signal to a constant value
  In1 : Inport
  Multiport Switch : MultiPortSwitch  DataPortOrder=Zero-based contiguous  Inputs=2  zeroidx=on
  Override Value : Constant  Value=0  OutDataTypeStr=double
  Signal Override Switch 0 = Use Model 1 = Use Constant : Constant  Value=0
  Out1 : Outport
  wires:
  Override Value/1 -> Multiport Switch/3
  Multiport Switch/1 -> Out1/1
  In1/1 -> Multiport Switch/2
  Signal Override Switch 0 = Use Model 1 = Use Constant/1 -> Multiport Switch/1

== system P2_SIL_Model_Diag/Controller/HSC/Camaro Fault Detection/Input Conversions/DriverInput_Conversions/Override V [mph] ==
  note: This subsystem is used to override the model value of a signal to a constant value
  note: Override Switch Subsystem
  In1 : Inport
  Multiport Switch : MultiPortSwitch  DataPortOrder=Zero-based contiguous  Inputs=2  zeroidx=on
  Override Value : Constant  Value=0  OutDataTypeStr=double
  Signal Override Switch 0 = Use Model 1 = Use Constant : Constant  Value=0
  Out1 : Outport
  wires:
  Signal Override Switch 0 = Use Model 1 = Use Constant/1 -> Multiport Switch/1
  In1/1 -> Multiport Switch/2
  Multiport Switch/1 -> Out1/1
  Override Value/1 -> Multiport Switch/3

== system P2_SIL_Model_Diag/Controller/HSC/Camaro Fault Detection/Input Conversions/ECM_Conversions/Override  ECMrollingAliveCnt ==
  note: Override Switch Subsystem
  note: This subsystem is used to override the model value of a signal to a constant value
  In1 : Inport
  Multiport Switch : MultiPortSwitch  DataPortOrder=Zero-based contiguous  Inputs=2  zeroidx=on
  Override Value : Constant  Value=0  OutDataTypeStr=double
  Signal Override Switch 0 = Use Model 1 = Use Constant : Constant  Value=0
  Out1 : Outport
  wires:
  Override Value/1 -> Multiport Switch/3
  Multiport Switch/1 -> Out1/1
  In1/1 -> Multiport Switch/2
  Signal Override Switch 0 = Use Model 1 = Use Constant/1 -> Multiport Switch/1

== system P2_SIL_Model_Diag/Controller/HSC/Camaro Fault Detection/Input Conversions/ECM_Conversions/Override  EngActStdyStTorq_Nm ==
  note: Override Switch Subsystem
  note: This subsystem is used to override the model value of a signal to a constant value
  In1 : Inport
  Multiport Switch : MultiPortSwitch  DataPortOrder=Zero-based contiguous  Inputs=2  zeroidx=on
  Override Value : Constant  Value=0  OutDataTypeStr=double
  Signal Override Switch 0 = Use Model 1 = Use Constant : Constant  Value=0
  Out1 : Outport
  wires:
  Override Value/1 -> Multiport Switch/3
  Multiport Switch/1 -> Out1/1
  In1/1 -> Multiport Switch/2
  Signal Override Switch 0 = Use Model 1 = Use Constant/1 -> Multiport Switch/1

== system P2_SIL_Model_Diag/Controller/HSC/Camaro Fault Detection/Input Conversions/ECM_Conversions/Override  EngRunAtv ==
  note: This subsystem is used to override the model value of a signal to a constant value
  note: Override Switch Subsystem
  In1 : Inport
  Multiport Switch : MultiPortSwitch  DataPortOrder=Zero-based contiguous  Inputs=2  zeroidx=on
  Override Value : Constant  Value=0  OutDataTypeStr=double
  Signal Override Switch 0 = Use Model 1 = Use Constant : Constant  Value=0
  Out1 : Outport
  wires:
  Signal Override Switch 0 = Use Model 1 = Use Constant/1 -> Multiport Switch/1
  In1/1 -> Multiport Switch/2
  Multiport Switch/1 -> Out1/1
  Override Value/1 -> Multiport Switch/3

== system P2_SIL_Model_Diag/Controller/HSC/Camaro Fault Detection/Input Conversions/ECM_Conversions/Override  Engine_Temp[DegC] ==
  note: Override Switch Subsystem
  note: This subsystem is used to override the model value of a signal to a constant value
  In1 : Inport
  Multiport Switch : MultiPortSwitch  DataPortOrder=Zero-based contiguous  Inputs=2  zeroidx=on
  Override Value : Constant  Value=0  OutDataTypeStr=double
  Signal Override Switch 0 = Use Model 1 = Use Constant : Constant  Value=0
  Out1 : Outport
  wires:
  Override Value/1 -> Multiport Switch/3
  Multiport Switch/1 -> Out1/1
  In1/1 -> Multiport Switch/2
  Signal Override Switch 0 = Use Model 1 = Use Constant/1 -> Multiport Switch/1

== system P2_SIL_Model_Diag/Controller/HSC/Camaro Fault Detection/Input Conversions/MCU_Conversions/Override  DC_Bus_Voltage ==
  note: This subsystem is used to override the model value of a signal to a constant value
  note: Override Switch Subsystem
  In1 : Inport
  Multiport Switch : MultiPortSwitch  DataPortOrder=Zero-based contiguous  Inputs=2  zeroidx=on
  Override Value : Constant  Value=0  OutDataTypeStr=double
  Signal Override Switch 0 = Use Model 1 = Use Constant : Constant  Value=0
  Out1 : Outport
  wires:
  Signal Override Switch 0 = Use Model 1 = Use Constant/1 -> Multiport Switch/1
  In1/1 -> Multiport Switch/2
  Multiport Switch/1 -> Out1/1
  Override Value/1 -> Multiport Switch/3

== system P2_SIL_Model_Diag/Controller/HSC/Camaro Fault Detection/Input Conversions/MCU_Conversions/Override  Direction_feedback ==
  note: This subsystem is used to override the model value of a signal to a constant value
  note: Override Switch Subsystem
  In1 : Inport
  Multiport Switch : MultiPortSwitch  DataPortOrder=Zero-based contiguous  Inputs=2  zeroidx=on
  Override Value : Constant  Value=0  OutDataTypeStr=double
  Signal Override Switch 0 = Use Model 1 = Use Constant : Constant  Value=0
  Out1 : Outport
  wires:
  Signal Override Switch 0 = Use Model 1 = Use Constant/1 -> Multiport Switch/1
  In1/1 -> Multiport Switch/2
  Multiport Switch/1 -> Out1/1
  Override Value/1 -> Multiport Switch/3

== system P2_SIL_Model_Diag/Controller/HSC/Camaro Fault Detection/Input Conversions/MCU_Conversions/Override  Inverter_enable_state ==
  note: Override Switch Subsystem
  note: This subsystem is used to override the model value of a signal to a constant value
  In1 : Inport
  Multiport Switch : MultiPortSwitch  DataPortOrder=Zero-based contiguous  Inputs=2  zeroidx=on
  Override Value : Constant  Value=0  OutDataTypeStr=double
  Signal Override Switch 0 = Use Model 1 = Use Constant : Constant  Value=0
  Out1 : Outport
  wires:
  Override Value/1 -> Multiport Switch/3
  Multiport Switch/1 -> Out1/1
  In1/1 -> Multiport Switch/2
  Signal Override Switch 0 = Use Model 1 = Use Constant/1 -> Multiport Switch/1

== system P2_SIL_Model_Diag/Controller/HSC/Camaro Fault Detection/Input Conversions/MCU_Conversions/Override  Motor_Direction ==
  note: Override Switch Subsystem
  note: This subsystem is used to override the model value of a signal to a constant value
  In1 : Inport
  Multiport Switch : MultiPortSwitch  DataPortOrder=Zero-based contiguous  Inputs=2  zeroidx=on
  Override Value : Constant  Value=0  OutDataTypeStr=double
  Signal Override Switch 0 = Use Model 1 = Use Constant : Constant  Value=0
  Out1 : Outport
  wires:
  Override Value/1 -> Multiport Switch/3
  Multiport Switch/1 -> Out1/1
  In1/1 -> Multiport Switch/2
  Signal Override Switch 0 = Use Model 1 = Use Constant/1 -> Multiport Switch/1

== system P2_SIL_Model_Diag/Controller/HSC/Camaro Fault Detection/Input Conversions/MCU_Conversions/Override  Torq_Feedback ==
  note: Override Switch Subsystem
  note: This subsystem is used to override the model value of a signal to a constant value
  In1 : Inport
  Multiport Switch : MultiPortSwitch  DataPortOrder=Zero-based contiguous  Inputs=2  zeroidx=on
  Override Value : Constant  Value=0  OutDataTypeStr=double
  Signal Override Switch 0 = Use Model 1 = Use Constant : Constant  Value=0
  Out1 : Outport
  wires:
  Override Value/1 -> Multiport Switch/3
  Multiport Switch/1 -> Out1/1
  In1/1 -> Multiport Switch/2
  Signal Override Switch 0 = Use Model 1 = Use Constant/1 -> Multiport Switch/1
